simulink model "ExtraCredit"  (R2016a)
settings: Solver=VariableStepAuto  StartTime=0.0  StopTime=10.0  RelTol=1e-3
libraries: hdlsllib x17
(part 1 of 2)
settings Model: Creator=duyvu  LastModifiedBy=duyvu

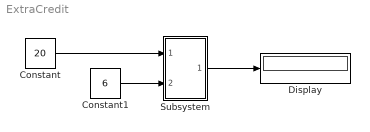
== system ExtraCredit ==
  Constant : Constant  Value=20  OutDataTypeStr=int8
  Constant1 : Constant  Value=6  OutDataTypeStr=int8
  Display : Display
  Subsystem : Subsystem
  wires:
  Subsystem/1(Result) -> Display/1
  Constant/1 -> Subsystem/1(Number1)
  Constant1/1 -> Subsystem/2(Number2)

== system ExtraCredit/Subsystem ==
  Number1 : Inport  OutDataTypeStr=int8
  Number2 : Inport  Port=2  OutDataTypeStr=int8
  Subsystem : Subsystem
  Result : Outport  OutDataTypeStr=int16
  wires:
  Number1/1 -> Subsystem/1(Number1)
  Number2/1 -> Subsystem/2(Number2)
  Subsystem/1(Result) -> Result/1

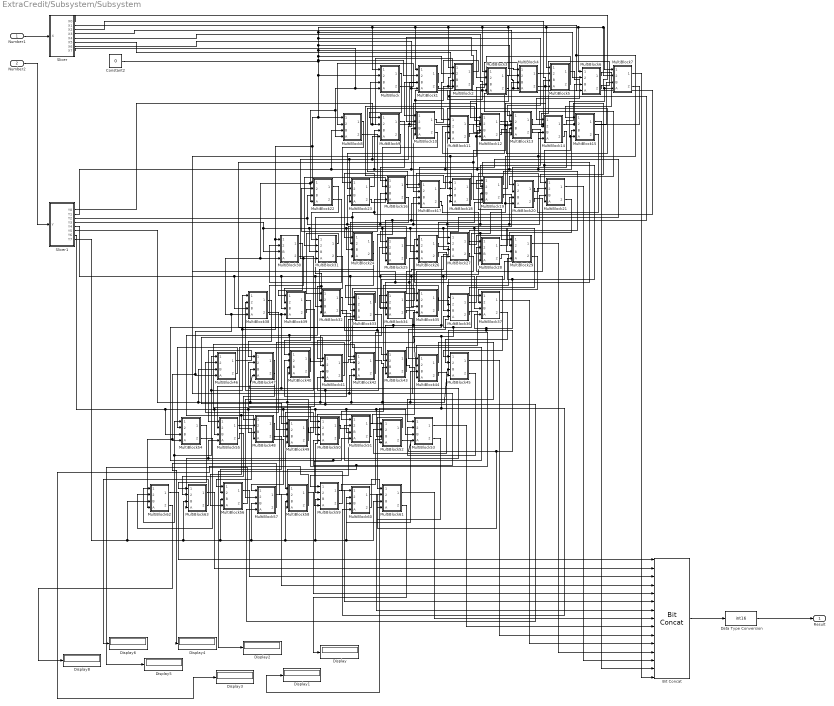
== system ExtraCredit/Subsystem/Subsystem ==
  Number1 : Inport  OutDataTypeStr=int8
  Number2 : Inport  Port=2  OutDataTypeStr=int8
  Bit Concat : hdlsllib/HDL Operations/Bit Concat  numInputs=15
  Constant2 : Constant  Value=0  OutDataTypeStr=boolean
  Data Type Conversion : DataTypeConversion  OutDataTypeStr=int16  ConvertRealWorld=Stored Integer (SI)
  Display{,1..6,8} (8 alike) : Display
      Display settings: Format=binary (Stored Integer)
      Display1 settings: Format=binary (Stored Integer)
  MultiBlock : Subsystem
  MultiBlock1 : Subsystem
  MultiBlock10 : Subsystem
  MultiBlock11 : Subsystem
  MultiBlock12 : Subsystem
  MultiBlock13 : Subsystem
  MultiBlock14 : Subsystem
  MultiBlock15 : Subsystem
  MultiBlock16 : Subsystem
  MultiBlock17 : Subsystem
  MultiBlock18 : Subsystem
  MultiBlock19 : Subsystem
  MultiBlock2 : Subsystem
  MultiBlock20 : Subsystem
  MultiBlock21 : Subsystem
  MultiBlock22 : Subsystem
  MultiBlock23 : Subsystem
  MultiBlock24 : Subsystem
  MultiBlock25 : Subsystem
  MultiBlock26 : Subsystem
  MultiBlock27 : Subsystem
  MultiBlock28 : Subsystem
  MultiBlock29 : Subsystem
  MultiBlock3 : Subsystem
  MultiBlock30 : Subsystem
  MultiBlock31 : Subsystem
  MultiBlock32 : Subsystem
  MultiBlock33 : Subsystem
  MultiBlock34 : Subsystem
  MultiBlock35 : Subsystem
  MultiBlock36 : Subsystem
  MultiBlock37 : Subsystem
  MultiBlock38 : Subsystem
  MultiBlock39 : Subsystem
  MultiBlock4 : Subsystem
  MultiBlock40 : Subsystem
  MultiBlock41 : Subsystem
  MultiBlock42 : Subsystem
  MultiBlock43 : Subsystem
  MultiBlock44 : Subsystem
  MultiBlock45 : Subsystem
  MultiBlock46 : Subsystem
  MultiBlock47 : Subsystem
  MultiBlock48 : Subsystem
  MultiBlock49 : Subsystem
  MultiBlock5 : Subsystem
  MultiBlock50 : Subsystem
  MultiBlock51 : Subsystem
  MultiBlock52 : Subsystem
  MultiBlock53 : Subsystem
  MultiBlock54 : Subsystem
  MultiBlock55 : Subsystem
  MultiBlock56 : Subsystem
  MultiBlock57 : Subsystem
  MultiBlock58 : Subsystem
  MultiBlock59 : Subsystem
  MultiBlock6 : Subsystem
  MultiBlock60 : Subsystem
  MultiBlock61 : Subsystem
  MultiBlock62 : Subsystem
  MultiBlock63 : Subsystem
  MultiBlock7 : Subsystem
  MultiBlock8 : Subsystem
  MultiBlock9 : Subsystem
  Slicer : Subsystem
  Slicer1 : Subsystem
  Result : Outport  OutDataTypeStr=int16
  wires:
  MultiBlock15/2(Carry) -> MultiBlock21/2(Cin)
  MultiBlock3/1(Sum) -> MultiBlock12/1(SumIn)
  Slicer1/1(Y0) -> MultiBlock/3(B), MultiBlock1/3(B), MultiBlock2/3(B), MultiBlock3/3(B), MultiBlock4/3(B), MultiBlock5/3(B), MultiBlock6/3(B), MultiBlock7/3(B)
  MultiBlock6/1(Sum) -> MultiBlock15/1(SumIn)
  MultiBlock12/1(Sum) -> MultiBlock19/1(SumIn)
  MultiBlock5/1(Sum) -> MultiBlock14/1(SumIn)
  MultiBlock/1(Sum) -> MultiBlock9/1(SumIn)
  MultiBlock4/1(Sum) -> MultiBlock13/1(SumIn)
  MultiBlock2/2(Carry) -> MultiBlock10/2(Cin)
  MultiBlock10/2(Carry) -> MultiBlock16/2(Cin)
  MultiBlock2/1(Sum) -> MultiBlock11/1(SumIn)
  MultiBlock1/1(Sum) -> MultiBlock10/1(SumIn)
  MultiBlock12/2(Carry) -> MultiBlock18/2(Cin)
  MultiBlock62/1(Sum) -> Bit Concat/1
  MultiBlock60/1(Sum) -> Bit Concat/7
  MultiBlock13/2(Carry) -> MultiBlock19/2(Cin)
  MultiBlock14/2(Carry) -> MultiBlock20/2(Cin)
  MultiBlock63/1(Sum) -> Bit Concat/2
  MultiBlock6/2(Carry) -> MultiBlock14/2(Cin)
  MultiBlock58/1(Sum) -> Bit Concat/5
  MultiBlock56/1(Sum) -> Bit Concat/3
  MultiBlock5/2(Carry) -> MultiBlock13/2(Cin)
  MultiBlock15/1(Sum) -> Bit Concat/14
  Slicer1/7(Y6) -> MultiBlock54/3(B), MultiBlock55/3(B), MultiBlock48/3(B), MultiBlock49/3(B), MultiBlock50/3(B), MultiBlock51/3(B), MultiBlock52/3(B), MultiBlock53/3(B)
  MultiBlock4/2(Carry) -> MultiBlock12/2(Cin)
  MultiBlock7/2(Carry) -> MultiBlock15/2(Cin)
  MultiBlock52/2(Carry) -> MultiBlock60/2(Cin)
  MultiBlock21/2(Carry) -> MultiBlock29/2(Cin)
  MultiBlock49/2(Carry) -> MultiBlock57/2(Cin)
  MultiBlock34/2(Carry) -> MultiBlock42/2(Cin)
  MultiBlock42/2(Carry) -> MultiBlock50/2(Cin)
  MultiBlock33/2(Carry) -> MultiBlock41/2(Cin)
  MultiBlock22/1(Sum) -> MultiBlock31/1(SumIn)
  MultiBlock16/1(Sum) -> MultiBlock25/1(SumIn)
  MultiBlock32/2(Carry) -> MultiBlock40/2(Cin)
  MultiBlock41/2(Carry) -> MultiBlock49/2(Cin)
  MultiBlock39/2(Carry) -> MultiBlock47/2(Cin)
  MultiBlock57/2(Carry) -> Display4/1
  MultiBlock30/1(Sum) -> MultiBlock39/1(SumIn)
  MultiBlock31/1(Sum) -> MultiBlock32/1(SumIn)
  MultiBlock55/2(Carry) -> MultiBlock63/2(Cin)
  MultiBlock24/2(Carry) -> MultiBlock32/2(Cin)
  MultiBlock59/2(Carry) -> Display2/1
  MultiBlock20/2(Carry) -> MultiBlock28/2(Cin)
  MultiBlock31/2(Carry) -> MultiBlock39/2(Cin)
  MultiBlock28/1(Sum) -> MultiBlock37/1(SumIn)
  MultiBlock36/1(Sum) -> MultiBlock45/1(SumIn)
  MultiBlock25/2(Carry) -> MultiBlock33/2(Cin)
  MultiBlock34/1(Sum) -> MultiBlock43/1(SumIn)
  MultiBlock45/2(Carry) -> MultiBlock53/2(Cin)
  MultiBlock10/1(Sum) -> MultiBlock17/1(SumIn)
  MultiBlock61/2(Carry) -> Display/1
  MultiBlock38/2(Carry) -> MultiBlock46/2(Cin)
  MultiBlock17/2(Carry) -> MultiBlock25/2(Cin)
  MultiBlock19/2(Carry) -> MultiBlock27/2(Cin)
  MultiBlock43/1(Sum) -> MultiBlock52/1(SumIn)
  MultiBlock44/1(Sum) -> MultiBlock53/1(SumIn)
  MultiBlock52/1(Sum) -> MultiBlock61/1(SumIn)
  MultiBlock46/2(Carry) -> MultiBlock54/2(Cin)
  MultiBlock47/2(Carry) -> MultiBlock55/2(Cin)
  MultiBlock9/1(Sum) -> MultiBlock16/1(SumIn)
  MultiBlock18/2(Carry) -> MultiBlock26/2(Cin)
  MultiBlock56/2(Carry) -> Display5/1
  MultiBlock8/1(Sum) -> MultiBlock23/1(SumIn)
  MultiBlock32/1(Sum) -> MultiBlock41/1(SumIn)
  MultiBlock58/2(Carry) -> Display3/1
  MultiBlock35/1(Sum) -> MultiBlock44/1(SumIn)
  MultiBlock51/2(Carry) -> MultiBlock59/2(Cin)
  MultiBlock16/2(Carry) -> MultiBlock24/2(Cin)
  MultiBlock30/2(Carry) -> MultiBlock38/2(Cin)
  MultiBlock22/2(Carry) -> MultiBlock30/2(Cin)
  MultiBlock47/1(Sum) -> MultiBlock48/1(SumIn)
  MultiBlock44/2(Carry) -> MultiBlock52/2(Cin)
  MultiBlock50/2(Carry) -> MultiBlock58/2(Cin)
  MultiBlock39/1(Sum) -> MultiBlock40/1(SumIn)
  MultiBlock41/1(Sum) -> MultiBlock50/1(SumIn)
  MultiBlock42/1(Sum) -> MultiBlock51/1(SumIn)
  MultiBlock37/2(Carry) -> MultiBlock45/2(Cin)
  MultiBlock50/1(Sum) -> MultiBlock59/1(SumIn)
  MultiBlock23/2(Carry) -> MultiBlock31/2(Cin)
  MultiBlock25/1(Sum) -> MultiBlock34/1(SumIn)
  MultiBlock27/1(Sum) -> MultiBlock36/1(SumIn)
  MultiBlock38/1(Sum) -> MultiBlock47/1(SumIn)
  MultiBlock20/1(Sum) -> MultiBlock29/1(SumIn)
  MultiBlock18/1(Sum) -> MultiBlock27/1(SumIn)
  MultiBlock19/1(Sum) -> MultiBlock28/1(SumIn)
  MultiBlock17/1(Sum) -> MultiBlock26/1(SumIn)
  MultiBlock24/1(Sum) -> MultiBlock33/1(SumIn)
  MultiBlock35/2(Carry) -> MultiBlock43/2(Cin)
  MultiBlock43/2(Carry) -> MultiBlock51/2(Cin)
  MultiBlock54/1(Sum) -> MultiBlock63/1(SumIn)
  MultiBlock40/1(Sum) -> MultiBlock49/1(SumIn)
  MultiBlock54/2(Carry) -> MultiBlock62/2(Cin)
  MultiBlock40/2(Carry) -> MultiBlock48/2(Cin)
  MultiBlock55/1(Sum) -> MultiBlock56/1(SumIn)
  MultiBlock48/2(Carry) -> MultiBlock56/2(Cin)
  MultiBlock51/1(Sum) -> MultiBlock60/1(SumIn)
  MultiBlock26/1(Sum) -> MultiBlock35/1(SumIn)
  MultiBlock53/2(Carry) -> MultiBlock61/2(Cin)
  MultiBlock33/1(Sum) -> MultiBlock42/1(SumIn)
  Slicer/8(X7) -> MultiBlock30/4(A), MultiBlock62/4(A), MultiBlock54/4(A), MultiBlock46/4(A), MultiBlock38/4(A), MultiBlock22/4(A), MultiBlock8/4(A), MultiBlock/4(A)
  Slicer/4(X3) -> MultiBlock26/4(A), MultiBlock58/4(A), MultiBlock50/4(A), MultiBlock42/4(A), MultiBlock34/4(A), MultiBlock18/4(A), MultiBlock12/4(A), MultiBlock4/4(A)
  Slicer/5(X4) -> MultiBlock33/4(A), MultiBlock49/4(A), MultiBlock57/4(A), MultiBlock41/4(A), MultiBlock25/4(A), MultiBlock17/4(A), MultiBlock11/4(A), MultiBlock3/4(A)
  MultiBlock36/2(Carry) -> MultiBlock44/2(Cin)
  MultiBlock46/1(Sum) -> MultiBlock55/1(SumIn)
  Slicer1/4(Y3) -> MultiBlock30/3(B), MultiBlock31/3(B), MultiBlock24/3(B), MultiBlock25/3(B), MultiBlock26/3(B), MultiBlock27/3(B), MultiBlock28/3(B), MultiBlock29/3(B)
  Slicer/3(X2) -> MultiBlock5/4(A), MultiBlock19/4(A), MultiBlock27/4(A), MultiBlock59/4(A), MultiBlock51/4(A), MultiBlock43/4(A), MultiBlock35/4(A), MultiBlock13/4(A)
  Slicer/6(X5) -> MultiBlock56/4(A), MultiBlock48/4(A), MultiBlock40/4(A), MultiBlock32/4(A), MultiBlock24/4(A), MultiBlock16/4(A), MultiBlock10/4(A), MultiBlock2/4(A)
  Slicer/1(X0) -> MultiBlock45/4(A), MultiBlock61/4(A), MultiBlock53/4(A), MultiBlock37/4(A), MultiBlock29/4(A), MultiBlock21/4(A), MultiBlock15/4(A), MultiBlock7/4(A)
  Slicer/7(X6) -> MultiBlock47/4(A), MultiBlock63/4(A), MultiBlock55/4(A), MultiBlock39/4(A), MultiBlock31/4(A), MultiBlock23/4(A), MultiBlock9/4(A), MultiBlock1/4(A)
  Slicer/2(X1) -> MultiBlock6/4(A), MultiBlock44/4(A), MultiBlock52/4(A), MultiBlock60/4(A), MultiBlock36/4(A), MultiBlock28/4(A), MultiBlock20/4(A), MultiBlock14/4(A)
  MultiBlock26/2(Carry) -> MultiBlock34/2(Cin)
  Slicer1/6(Y5) -> MultiBlock46/3(B), MultiBlock47/3(B), MultiBlock40/3(B), MultiBlock41/3(B), MultiBlock42/3(B), MultiBlock43/3(B), MultiBlock44/3(B), MultiBlock45/3(B)
  MultiBlock13/1(Sum) -> MultiBlock20/1(SumIn)
  MultiBlock8/2(Carry) -> MultiBlock22/2(Cin)
  Slicer1/3(Y2) -> MultiBlock23/3(B), MultiBlock18/3(B), MultiBlock19/3(B), MultiBlock20/3(B), MultiBlock21/3(B), MultiBlock17/3(B), MultiBlock16/3(B), MultiBlock22/3(B)
  Number1/1 -> Slicer/1(X)
  Number2/1 -> Slicer1/1(Y)
  Slicer1/2(Y1) -> MultiBlock9/3(B), MultiBlock10/3(B), MultiBlock11/3(B), MultiBlock12/3(B), MultiBlock13/3(B), MultiBlock14/3(B), MultiBlock15/3(B), MultiBlock8/3(B)
  MultiBlock29/1(Sum) -> Bit Concat/12
  MultiBlock61/1(Sum) -> Bit Concat/8
  MultiBlock21/1(Sum) -> Bit Concat/13
  MultiBlock28/2(Carry) -> MultiBlock36/2(Cin)
  MultiBlock27/2(Carry) -> MultiBlock35/2(Cin)
  MultiBlock29/2(Carry) -> MultiBlock37/2(Cin)
  MultiBlock37/1(Sum) -> Bit Concat/11
  Constant2/1 -> MultiBlock/1(SumIn), MultiBlock1/1(SumIn), MultiBlock6/1(SumIn), MultiBlock7/1(SumIn), MultiBlock7/2(Cin), MultiBlock5/1(SumIn), MultiBlock4/1(SumIn), MultiBlock3/1(SumIn), MultiBlock2/1(SumIn), MultiBlock6/2(Cin), MultiBlock5/2(Cin), MultiBlock4/2(Cin), MultiBlock3/2(Cin), MultiBlock2/2(Cin), MultiBlock1/2(Cin), MultiBlock38/1(SumIn), MultiBlock46/1(SumIn), MultiBlock54/1(SumIn), MultiBlock62/1(SumIn), MultiBlock30/1(SumIn), MultiBlock22/1(SumIn), MultiBlock8/1(SumIn), MultiBlock/2(Cin)
  MultiBlock53/1(Sum) -> Bit Concat/9
  MultiBlock45/1(Sum) -> Bit Concat/10
  MultiBlock23/1(Sum) -> MultiBlock24/1(SumIn)
  MultiBlock59/1(Sum) -> Bit Concat/6
  Slicer1/8(Y7) -> MultiBlock62/3(B), MultiBlock63/3(B), MultiBlock56/3(B), MultiBlock57/3(B), MultiBlock58/3(B), MultiBlock59/3(B), MultiBlock61/3(B), MultiBlock60/3(B)
  MultiBlock48/1(Sum) -> MultiBlock57/1(SumIn)
  MultiBlock57/1(Sum) -> Bit Concat/4
  MultiBlock62/2(Carry) -> Display8/1
  Bit Concat/1 -> Data Type Conversion/1
  MultiBlock/2(Carry) -> MultiBlock8/2(Cin)
  Data Type Conversion/1 -> Result/1
  MultiBlock49/1(Sum) -> MultiBlock58/1(SumIn)
  MultiBlock63/2(Carry) -> Display6/1
  MultiBlock3/2(Carry) -> MultiBlock11/2(Cin)
  MultiBlock1/2(Carry) -> MultiBlock9/2(Cin)
  Slicer1/5(Y4) -> MultiBlock38/3(B), MultiBlock39/3(B), MultiBlock32/3(B), MultiBlock33/3(B), MultiBlock34/3(B), MultiBlock35/3(B), MultiBlock36/3(B), MultiBlock37/3(B)
  MultiBlock60/2(Carry) -> Display1/1
  MultiBlock7/1(Sum) -> Bit Concat/15
  MultiBlock11/2(Carry) -> MultiBlock17/2(Cin)
  MultiBlock9/2(Carry) -> MultiBlock23/2(Cin)
  MultiBlock11/1(Sum) -> MultiBlock18/1(SumIn)
  MultiBlock14/1(Sum) -> MultiBlock21/1(SumIn)

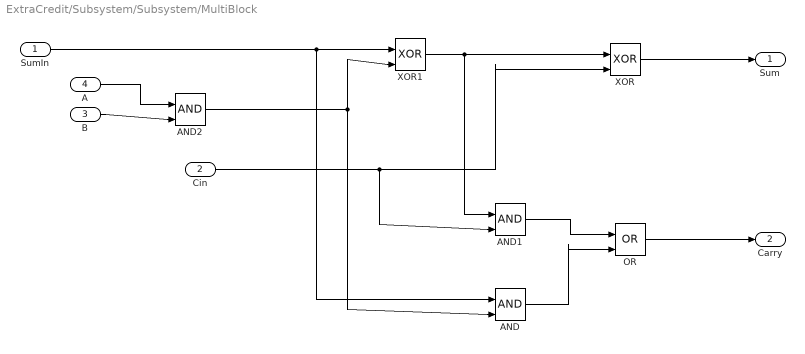
== system ExtraCredit/Subsystem/Subsystem/MultiBlock ==
  SumIn : Inport
  Cin : Inport  Port=2
  B : Inport  Port=3
  A : Inport  Port=4
  AND : Logic  IconShape=distinctive  AllPortsSameDT=off  OutDataTypeStr=boolean
  AND1 : Logic  IconShape=distinctive  AllPortsSameDT=off  OutDataTypeStr=boolean
  AND2 : Logic  IconShape=distinctive  AllPortsSameDT=off  OutDataTypeStr=boolean
  "OR " : Logic  Operator=OR  IconShape=distinctive  AllPortsSameDT=off  OutDataTypeStr=boolean
  XOR : Logic  Operator=XOR  IconShape=distinctive  AllPortsSameDT=off  OutDataTypeStr=boolean
  XOR1 : Logic  Operator=XOR  IconShape=distinctive  AllPortsSameDT=off  OutDataTypeStr=boolean
  Sum : Outport
  Carry : Outport  Port=2
  wires:
  SumIn/1 -> XOR1/1, AND/1
  XOR1/1 -> AND1/1, XOR/1
  Cin/1 -> XOR/2, AND1/2
  XOR/1 -> Sum/1
  AND2/1 -> AND/2, XOR1/2
  "OR "/1 -> Carry/1
  AND1/1 -> "OR "/1
  AND/1 -> "OR "/2
  B/1 -> AND2/2
  A/1 -> AND2/1

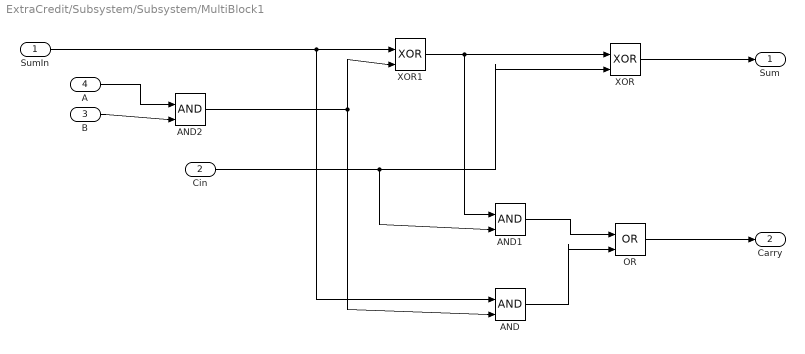
== system ExtraCredit/Subsystem/Subsystem/MultiBlock1 ==
  SumIn : Inport
  Cin : Inport  Port=2
  B : Inport  Port=3
  A : Inport  Port=4
  AND : Logic  IconShape=distinctive  AllPortsSameDT=off  OutDataTypeStr=boolean
  AND1 : Logic  IconShape=distinctive  AllPortsSameDT=off  OutDataTypeStr=boolean
  AND2 : Logic  IconShape=distinctive  AllPortsSameDT=off  OutDataTypeStr=boolean
  "OR " : Logic  Operator=OR  IconShape=distinctive  AllPortsSameDT=off  OutDataTypeStr=boolean
  XOR : Logic  Operator=XOR  IconShape=distinctive  AllPortsSameDT=off  OutDataTypeStr=boolean
  XOR1 : Logic  Operator=XOR  IconShape=distinctive  AllPortsSameDT=off  OutDataTypeStr=boolean
  Sum : Outport
  Carry : Outport  Port=2
  wires:
  SumIn/1 -> XOR1/1, AND/1
  XOR1/1 -> AND1/1, XOR/1
  Cin/1 -> XOR/2, AND1/2
  XOR/1 -> Sum/1
  AND2/1 -> AND/2, XOR1/2
  "OR "/1 -> Carry/1
  AND1/1 -> "OR "/1
  AND/1 -> "OR "/2
  B/1 -> AND2/2
  A/1 -> AND2/1

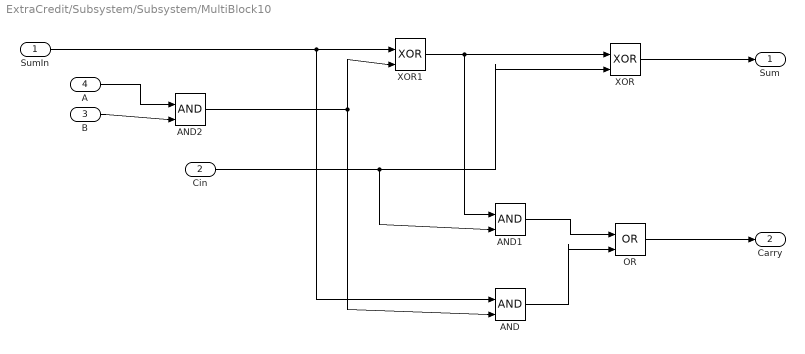
== system ExtraCredit/Subsystem/Subsystem/MultiBlock10 ==
  SumIn : Inport
  Cin : Inport  Port=2
  B : Inport  Port=3
  A : Inport  Port=4
  AND : Logic  IconShape=distinctive  AllPortsSameDT=off  OutDataTypeStr=boolean
  AND1 : Logic  IconShape=distinctive  AllPortsSameDT=off  OutDataTypeStr=boolean
  AND2 : Logic  IconShape=distinctive  AllPortsSameDT=off  OutDataTypeStr=boolean
  "OR " : Logic  Operator=OR  IconShape=distinctive  AllPortsSameDT=off  OutDataTypeStr=boolean
  XOR : Logic  Operator=XOR  IconShape=distinctive  AllPortsSameDT=off  OutDataTypeStr=boolean
  XOR1 : Logic  Operator=XOR  IconShape=distinctive  AllPortsSameDT=off  OutDataTypeStr=boolean
  Sum : Outport
  Carry : Outport  Port=2
  wires:
  SumIn/1 -> XOR1/1, AND/1
  XOR1/1 -> AND1/1, XOR/1
  Cin/1 -> XOR/2, AND1/2
  XOR/1 -> Sum/1
  AND2/1 -> AND/2, XOR1/2
  "OR "/1 -> Carry/1
  AND1/1 -> "OR "/1
  AND/1 -> "OR "/2
  B/1 -> AND2/2
  A/1 -> AND2/1

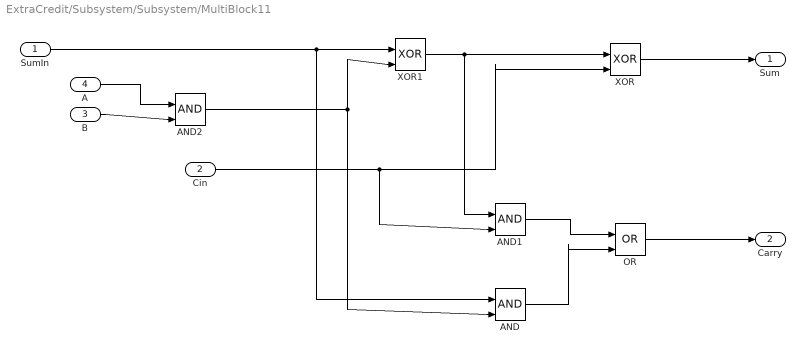
== system ExtraCredit/Subsystem/Subsystem/MultiBlock11 ==
  SumIn : Inport
  Cin : Inport  Port=2
  B : Inport  Port=3
  A : Inport  Port=4
  AND : Logic  IconShape=distinctive  AllPortsSameDT=off  OutDataTypeStr=boolean
  AND1 : Logic  IconShape=distinctive  AllPortsSameDT=off  OutDataTypeStr=boolean
  AND2 : Logic  IconShape=distinctive  AllPortsSameDT=off  OutDataTypeStr=boolean
  "OR " : Logic  Operator=OR  IconShape=distinctive  AllPortsSameDT=off  OutDataTypeStr=boolean
  XOR : Logic  Operator=XOR  IconShape=distinctive  AllPortsSameDT=off  OutDataTypeStr=boolean
  XOR1 : Logic  Operator=XOR  IconShape=distinctive  AllPortsSameDT=off  OutDataTypeStr=boolean
  Sum : Outport
  Carry : Outport  Port=2
  wires:
  SumIn/1 -> XOR1/1, AND/1
  XOR1/1 -> AND1/1, XOR/1
  Cin/1 -> XOR/2, AND1/2
  XOR/1 -> Sum/1
  AND2/1 -> AND/2, XOR1/2
  "OR "/1 -> Carry/1
  AND1/1 -> "OR "/1
  AND/1 -> "OR "/2
  B/1 -> AND2/2
  A/1 -> AND2/1

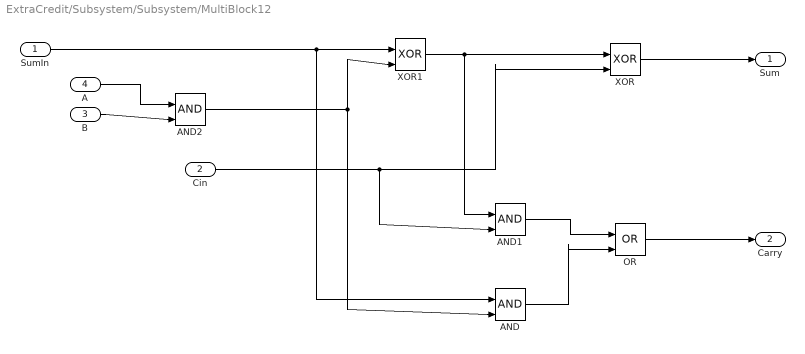
== system ExtraCredit/Subsystem/Subsystem/MultiBlock12 ==
  SumIn : Inport
  Cin : Inport  Port=2
  B : Inport  Port=3
  A : Inport  Port=4
  AND : Logic  IconShape=distinctive  AllPortsSameDT=off  OutDataTypeStr=boolean
  AND1 : Logic  IconShape=distinctive  AllPortsSameDT=off  OutDataTypeStr=boolean
  AND2 : Logic  IconShape=distinctive  AllPortsSameDT=off  OutDataTypeStr=boolean
  "OR " : Logic  Operator=OR  IconShape=distinctive  AllPortsSameDT=off  OutDataTypeStr=boolean
  XOR : Logic  Operator=XOR  IconShape=distinctive  AllPortsSameDT=off  OutDataTypeStr=boolean
  XOR1 : Logic  Operator=XOR  IconShape=distinctive  AllPortsSameDT=off  OutDataTypeStr=boolean
  Sum : Outport
  Carry : Outport  Port=2
  wires:
  SumIn/1 -> XOR1/1, AND/1
  XOR1/1 -> AND1/1, XOR/1
  Cin/1 -> XOR/2, AND1/2
  XOR/1 -> Sum/1
  AND2/1 -> AND/2, XOR1/2
  "OR "/1 -> Carry/1
  AND1/1 -> "OR "/1
  AND/1 -> "OR "/2
  B/1 -> AND2/2
  A/1 -> AND2/1

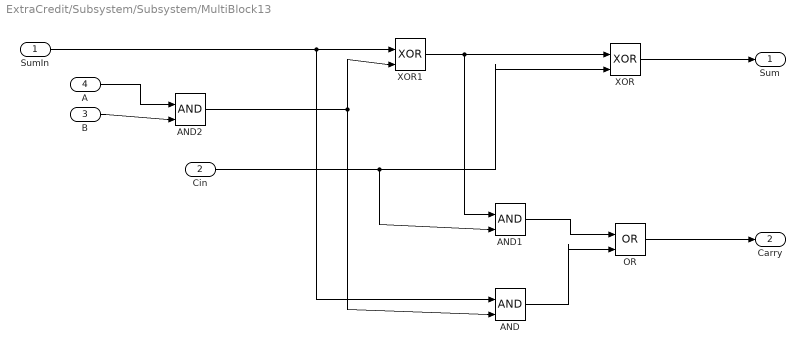
== system ExtraCredit/Subsystem/Subsystem/MultiBlock13 ==
  SumIn : Inport
  Cin : Inport  Port=2
  B : Inport  Port=3
  A : Inport  Port=4
  AND : Logic  IconShape=distinctive  AllPortsSameDT=off  OutDataTypeStr=boolean
  AND1 : Logic  IconShape=distinctive  AllPortsSameDT=off  OutDataTypeStr=boolean
  AND2 : Logic  IconShape=distinctive  AllPortsSameDT=off  OutDataTypeStr=boolean
  "OR " : Logic  Operator=OR  IconShape=distinctive  AllPortsSameDT=off  OutDataTypeStr=boolean
  XOR : Logic  Operator=XOR  IconShape=distinctive  AllPortsSameDT=off  OutDataTypeStr=boolean
  XOR1 : Logic  Operator=XOR  IconShape=distinctive  AllPortsSameDT=off  OutDataTypeStr=boolean
  Sum : Outport
  Carry : Outport  Port=2
  wires:
  SumIn/1 -> XOR1/1, AND/1
  XOR1/1 -> AND1/1, XOR/1
  Cin/1 -> XOR/2, AND1/2
  XOR/1 -> Sum/1
  AND2/1 -> AND/2, XOR1/2
  "OR "/1 -> Carry/1
  AND1/1 -> "OR "/1
  AND/1 -> "OR "/2
  B/1 -> AND2/2
  A/1 -> AND2/1

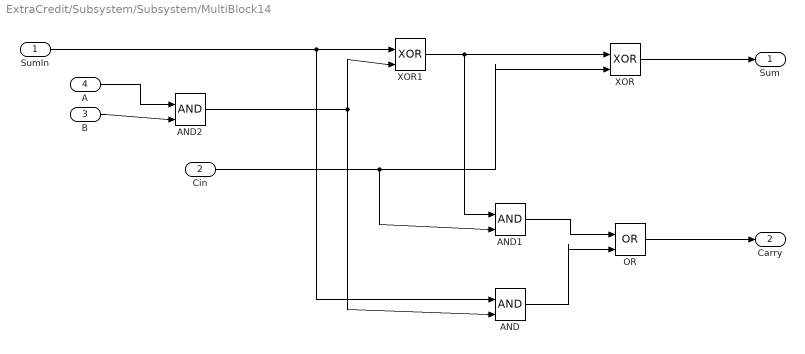
== system ExtraCredit/Subsystem/Subsystem/MultiBlock14 ==
  SumIn : Inport
  Cin : Inport  Port=2
  B : Inport  Port=3
  A : Inport  Port=4
  AND : Logic  IconShape=distinctive  AllPortsSameDT=off  OutDataTypeStr=boolean
  AND1 : Logic  IconShape=distinctive  AllPortsSameDT=off  OutDataTypeStr=boolean
  AND2 : Logic  IconShape=distinctive  AllPortsSameDT=off  OutDataTypeStr=boolean
  "OR " : Logic  Operator=OR  IconShape=distinctive  AllPortsSameDT=off  OutDataTypeStr=boolean
  XOR : Logic  Operator=XOR  IconShape=distinctive  AllPortsSameDT=off  OutDataTypeStr=boolean
  XOR1 : Logic  Operator=XOR  IconShape=distinctive  AllPortsSameDT=off  OutDataTypeStr=boolean
  Sum : Outport
  Carry : Outport  Port=2
  wires:
  SumIn/1 -> XOR1/1, AND/1
  XOR1/1 -> AND1/1, XOR/1
  Cin/1 -> XOR/2, AND1/2
  XOR/1 -> Sum/1
  AND2/1 -> AND/2, XOR1/2
  "OR "/1 -> Carry/1
  AND1/1 -> "OR "/1
  AND/1 -> "OR "/2
  B/1 -> AND2/2
  A/1 -> AND2/1

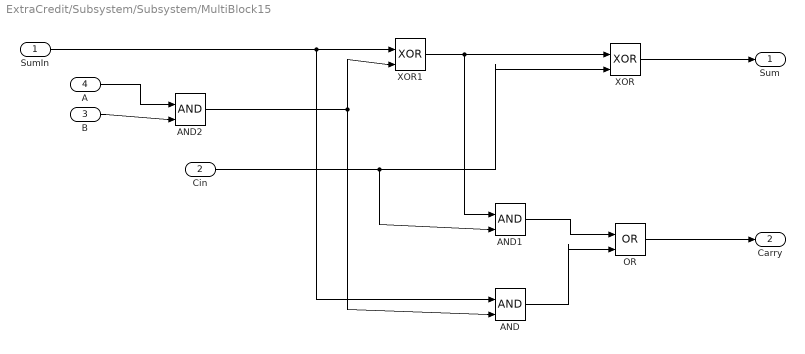
== system ExtraCredit/Subsystem/Subsystem/MultiBlock15 ==
  SumIn : Inport
  Cin : Inport  Port=2
  B : Inport  Port=3
  A : Inport  Port=4
  AND : Logic  IconShape=distinctive  AllPortsSameDT=off  OutDataTypeStr=boolean
  AND1 : Logic  IconShape=distinctive  AllPortsSameDT=off  OutDataTypeStr=boolean
  AND2 : Logic  IconShape=distinctive  AllPortsSameDT=off  OutDataTypeStr=boolean
  "OR " : Logic  Operator=OR  IconShape=distinctive  AllPortsSameDT=off  OutDataTypeStr=boolean
  XOR : Logic  Operator=XOR  IconShape=distinctive  AllPortsSameDT=off  OutDataTypeStr=boolean
  XOR1 : Logic  Operator=XOR  IconShape=distinctive  AllPortsSameDT=off  OutDataTypeStr=boolean
  Sum : Outport
  Carry : Outport  Port=2
  wires:
  SumIn/1 -> XOR1/1, AND/1
  XOR1/1 -> AND1/1, XOR/1
  Cin/1 -> XOR/2, AND1/2
  XOR/1 -> Sum/1
  AND2/1 -> AND/2, XOR1/2
  "OR "/1 -> Carry/1
  AND1/1 -> "OR "/1
  AND/1 -> "OR "/2
  B/1 -> AND2/2
  A/1 -> AND2/1

== system ExtraCredit/Subsystem/Subsystem/MultiBlock16 ==
  SumIn : Inport
  Cin : Inport  Port=2
  B : Inport  Port=3
  A : Inport  Port=4
  AND : Logic  IconShape=distinctive  AllPortsSameDT=off  OutDataTypeStr=boolean
  AND1 : Logic  IconShape=distinctive  AllPortsSameDT=off  OutDataTypeStr=boolean
  AND2 : Logic  IconShape=distinctive  AllPortsSameDT=off  OutDataTypeStr=boolean
  "OR " : Logic  Operator=OR  IconShape=distinctive  AllPortsSameDT=off  OutDataTypeStr=boolean
  XOR : Logic  Operator=XOR  IconShape=distinctive  AllPortsSameDT=off  OutDataTypeStr=boolean
  XOR1 : Logic  Operator=XOR  IconShape=distinctive  AllPortsSameDT=off  OutDataTypeStr=boolean
  Sum : Outport
  Carry : Outport  Port=2
  wires:
  SumIn/1 -> XOR1/1, AND/1
  XOR1/1 -> AND1/1, XOR/1
  Cin/1 -> XOR/2, AND1/2
  XOR/1 -> Sum/1
  AND2/1 -> AND/2, XOR1/2
  "OR "/1 -> Carry/1
  AND1/1 -> "OR "/1
  AND/1 -> "OR "/2
  B/1 -> AND2/2
  A/1 -> AND2/1

== system ExtraCredit/Subsystem/Subsystem/MultiBlock17 ==
  SumIn : Inport
  Cin : Inport  Port=2
  B : Inport  Port=3
  A : Inport  Port=4
  AND : Logic  IconShape=distinctive  AllPortsSameDT=off  OutDataTypeStr=boolean
  AND1 : Logic  IconShape=distinctive  AllPortsSameDT=off  OutDataTypeStr=boolean
  AND2 : Logic  IconShape=distinctive  AllPortsSameDT=off  OutDataTypeStr=boolean
  "OR " : Logic  Operator=OR  IconShape=distinctive  AllPortsSameDT=off  OutDataTypeStr=boolean
  XOR : Logic  Operator=XOR  IconShape=distinctive  AllPortsSameDT=off  OutDataTypeStr=boolean
  XOR1 : Logic  Operator=XOR  IconShape=distinctive  AllPortsSameDT=off  OutDataTypeStr=boolean
  Sum : Outport
  Carry : Outport  Port=2
  wires:
  SumIn/1 -> XOR1/1, AND/1
  XOR1/1 -> AND1/1, XOR/1
  Cin/1 -> XOR/2, AND1/2
  XOR/1 -> Sum/1
  AND2/1 -> AND/2, XOR1/2
  "OR "/1 -> Carry/1
  AND1/1 -> "OR "/1
  AND/1 -> "OR "/2
  B/1 -> AND2/2
  A/1 -> AND2/1

== system ExtraCredit/Subsystem/Subsystem/MultiBlock18 ==
  SumIn : Inport
  Cin : Inport  Port=2
  B : Inport  Port=3
  A : Inport  Port=4
  AND : Logic  IconShape=distinctive  AllPortsSameDT=off  OutDataTypeStr=boolean
  AND1 : Logic  IconShape=distinctive  AllPortsSameDT=off  OutDataTypeStr=boolean
  AND2 : Logic  IconShape=distinctive  AllPortsSameDT=off  OutDataTypeStr=boolean
  "OR " : Logic  Operator=OR  IconShape=distinctive  AllPortsSameDT=off  OutDataTypeStr=boolean
  XOR : Logic  Operator=XOR  IconShape=distinctive  AllPortsSameDT=off  OutDataTypeStr=boolean
  XOR1 : Logic  Operator=XOR  IconShape=distinctive  AllPortsSameDT=off  OutDataTypeStr=boolean
  Sum : Outport
  Carry : Outport  Port=2
  wires:
  SumIn/1 -> XOR1/1, AND/1
  XOR1/1 -> AND1/1, XOR/1
  Cin/1 -> XOR/2, AND1/2
  XOR/1 -> Sum/1
  AND2/1 -> AND/2, XOR1/2
  "OR "/1 -> Carry/1
  AND1/1 -> "OR "/1
  AND/1 -> "OR "/2
  B/1 -> AND2/2
  A/1 -> AND2/1

== system ExtraCredit/Subsystem/Subsystem/MultiBlock19 ==
  SumIn : Inport
  Cin : Inport  Port=2
  B : Inport  Port=3
  A : Inport  Port=4
  AND : Logic  IconShape=distinctive  AllPortsSameDT=off  OutDataTypeStr=boolean
  AND1 : Logic  IconShape=distinctive  AllPortsSameDT=off  OutDataTypeStr=boolean
  AND2 : Logic  IconShape=distinctive  AllPortsSameDT=off  OutDataTypeStr=boolean
  "OR " : Logic  Operator=OR  IconShape=distinctive  AllPortsSameDT=off  OutDataTypeStr=boolean
  XOR : Logic  Operator=XOR  IconShape=distinctive  AllPortsSameDT=off  OutDataTypeStr=boolean
  XOR1 : Logic  Operator=XOR  IconShape=distinctive  AllPortsSameDT=off  OutDataTypeStr=boolean
  Sum : Outport
  Carry : Outport  Port=2
  wires:
  SumIn/1 -> XOR1/1, AND/1
  XOR1/1 -> AND1/1, XOR/1
  Cin/1 -> XOR/2, AND1/2
  XOR/1 -> Sum/1
  AND2/1 -> AND/2, XOR1/2
  "OR "/1 -> Carry/1
  AND1/1 -> "OR "/1
  AND/1 -> "OR "/2
  B/1 -> AND2/2
  A/1 -> AND2/1

== system ExtraCredit/Subsystem/Subsystem/MultiBlock2 ==
  SumIn : Inport
  Cin : Inport  Port=2
  B : Inport  Port=3
  A : Inport  Port=4
  AND : Logic  IconShape=distinctive  AllPortsSameDT=off  OutDataTypeStr=boolean
  AND1 : Logic  IconShape=distinctive  AllPortsSameDT=off  OutDataTypeStr=boolean
  AND2 : Logic  IconShape=distinctive  AllPortsSameDT=off  OutDataTypeStr=boolean
  "OR " : Logic  Operator=OR  IconShape=distinctive  AllPortsSameDT=off  OutDataTypeStr=boolean
  XOR : Logic  Operator=XOR  IconShape=distinctive  AllPortsSameDT=off  OutDataTypeStr=boolean
  XOR1 : Logic  Operator=XOR  IconShape=distinctive  AllPortsSameDT=off  OutDataTypeStr=boolean
  Sum : Outport
  Carry : Outport  Port=2
  wires:
  SumIn/1 -> XOR1/1, AND/1
  XOR1/1 -> AND1/1, XOR/1
  Cin/1 -> XOR/2, AND1/2
  XOR/1 -> Sum/1
  AND2/1 -> AND/2, XOR1/2
  "OR "/1 -> Carry/1
  AND1/1 -> "OR "/1
  AND/1 -> "OR "/2
  B/1 -> AND2/2
  A/1 -> AND2/1

== system ExtraCredit/Subsystem/Subsystem/MultiBlock20 ==
  SumIn : Inport
  Cin : Inport  Port=2
  B : Inport  Port=3
  A : Inport  Port=4
  AND : Logic  IconShape=distinctive  AllPortsSameDT=off  OutDataTypeStr=boolean
  AND1 : Logic  IconShape=distinctive  AllPortsSameDT=off  OutDataTypeStr=boolean
  AND2 : Logic  IconShape=distinctive  AllPortsSameDT=off  OutDataTypeStr=boolean
  "OR " : Logic  Operator=OR  IconShape=distinctive  AllPortsSameDT=off  OutDataTypeStr=boolean
  XOR : Logic  Operator=XOR  IconShape=distinctive  AllPortsSameDT=off  OutDataTypeStr=boolean
  XOR1 : Logic  Operator=XOR  IconShape=distinctive  AllPortsSameDT=off  OutDataTypeStr=boolean
  Sum : Outport
  Carry : Outport  Port=2
  wires:
  SumIn/1 -> XOR1/1, AND/1
  XOR1/1 -> AND1/1, XOR/1
  Cin/1 -> XOR/2, AND1/2
  XOR/1 -> Sum/1
  AND2/1 -> AND/2, XOR1/2
  "OR "/1 -> Carry/1
  AND1/1 -> "OR "/1
  AND/1 -> "OR "/2
  B/1 -> AND2/2
  A/1 -> AND2/1

== system ExtraCredit/Subsystem/Subsystem/MultiBlock21 ==
  SumIn : Inport
  Cin : Inport  Port=2
  B : Inport  Port=3
  A : Inport  Port=4
  AND : Logic  IconShape=distinctive  AllPortsSameDT=off  OutDataTypeStr=boolean
  AND1 : Logic  IconShape=distinctive  AllPortsSameDT=off  OutDataTypeStr=boolean
  AND2 : Logic  IconShape=distinctive  AllPortsSameDT=off  OutDataTypeStr=boolean
  "OR " : Logic  Operator=OR  IconShape=distinctive  AllPortsSameDT=off  OutDataTypeStr=boolean
  XOR : Logic  Operator=XOR  IconShape=distinctive  AllPortsSameDT=off  OutDataTypeStr=boolean
  XOR1 : Logic  Operator=XOR  IconShape=distinctive  AllPortsSameDT=off  OutDataTypeStr=boolean
  Sum : Outport
  Carry : Outport  Port=2
  wires:
  SumIn/1 -> XOR1/1, AND/1
  XOR1/1 -> AND1/1, XOR/1
  Cin/1 -> XOR/2, AND1/2
  XOR/1 -> Sum/1
  AND2/1 -> AND/2, XOR1/2
  "OR "/1 -> Carry/1
  AND1/1 -> "OR "/1
  AND/1 -> "OR "/2
  B/1 -> AND2/2
  A/1 -> AND2/1

== system ExtraCredit/Subsystem/Subsystem/MultiBlock22 ==
  SumIn : Inport
  Cin : Inport  Port=2
  B : Inport  Port=3
  A : Inport  Port=4
  AND : Logic  IconShape=distinctive  AllPortsSameDT=off  OutDataTypeStr=boolean
  AND1 : Logic  IconShape=distinctive  AllPortsSameDT=off  OutDataTypeStr=boolean
  AND2 : Logic  IconShape=distinctive  AllPortsSameDT=off  OutDataTypeStr=boolean
  "OR " : Logic  Operator=OR  IconShape=distinctive  AllPortsSameDT=off  OutDataTypeStr=boolean
  XOR : Logic  Operator=XOR  IconShape=distinctive  AllPortsSameDT=off  OutDataTypeStr=boolean
  XOR1 : Logic  Operator=XOR  IconShape=distinctive  AllPortsSameDT=off  OutDataTypeStr=boolean
  Sum : Outport
  Carry : Outport  Port=2
  wires:
  SumIn/1 -> XOR1/1, AND/1
  XOR1/1 -> AND1/1, XOR/1
  Cin/1 -> XOR/2, AND1/2
  XOR/1 -> Sum/1
  AND2/1 -> AND/2, XOR1/2
  "OR "/1 -> Carry/1
  AND1/1 -> "OR "/1
  AND/1 -> "OR "/2
  B/1 -> AND2/2
  A/1 -> AND2/1

== system ExtraCredit/Subsystem/Subsystem/MultiBlock23 ==
  SumIn : Inport
  Cin : Inport  Port=2
  B : Inport  Port=3
  A : Inport  Port=4
  AND : Logic  IconShape=distinctive  AllPortsSameDT=off  OutDataTypeStr=boolean
  AND1 : Logic  IconShape=distinctive  AllPortsSameDT=off  OutDataTypeStr=boolean
  AND2 : Logic  IconShape=distinctive  AllPortsSameDT=off  OutDataTypeStr=boolean
  "OR " : Logic  Operator=OR  IconShape=distinctive  AllPortsSameDT=off  OutDataTypeStr=boolean
  XOR : Logic  Operator=XOR  IconShape=distinctive  AllPortsSameDT=off  OutDataTypeStr=boolean
  XOR1 : Logic  Operator=XOR  IconShape=distinctive  AllPortsSameDT=off  OutDataTypeStr=boolean
  Sum : Outport
  Carry : Outport  Port=2
  wires:
  SumIn/1 -> XOR1/1, AND/1
  XOR1/1 -> AND1/1, XOR/1
  Cin/1 -> XOR/2, AND1/2
  XOR/1 -> Sum/1
  AND2/1 -> AND/2, XOR1/2
  "OR "/1 -> Carry/1
  AND1/1 -> "OR "/1
  AND/1 -> "OR "/2
  B/1 -> AND2/2
  A/1 -> AND2/1

== system ExtraCredit/Subsystem/Subsystem/MultiBlock24 ==
  SumIn : Inport
  Cin : Inport  Port=2
  B : Inport  Port=3
  A : Inport  Port=4
  AND : Logic  IconShape=distinctive  AllPortsSameDT=off  OutDataTypeStr=boolean
  AND1 : Logic  IconShape=distinctive  AllPortsSameDT=off  OutDataTypeStr=boolean
  AND2 : Logic  IconShape=distinctive  AllPortsSameDT=off  OutDataTypeStr=boolean
  "OR " : Logic  Operator=OR  IconShape=distinctive  AllPortsSameDT=off  OutDataTypeStr=boolean
  XOR : Logic  Operator=XOR  IconShape=distinctive  AllPortsSameDT=off  OutDataTypeStr=boolean
  XOR1 : Logic  Operator=XOR  IconShape=distinctive  AllPortsSameDT=off  OutDataTypeStr=boolean
  Sum : Outport
  Carry : Outport  Port=2
  wires:
  SumIn/1 -> XOR1/1, AND/1
  XOR1/1 -> AND1/1, XOR/1
  Cin/1 -> XOR/2, AND1/2
  XOR/1 -> Sum/1
  AND2/1 -> AND/2, XOR1/2
  "OR "/1 -> Carry/1
  AND1/1 -> "OR "/1
  AND/1 -> "OR "/2
  B/1 -> AND2/2
  A/1 -> AND2/1

== system ExtraCredit/Subsystem/Subsystem/MultiBlock25 ==
  SumIn : Inport
  Cin : Inport  Port=2
  B : Inport  Port=3
  A : Inport  Port=4
  AND : Logic  IconShape=distinctive  AllPortsSameDT=off  OutDataTypeStr=boolean
  AND1 : Logic  IconShape=distinctive  AllPortsSameDT=off  OutDataTypeStr=boolean
  AND2 : Logic  IconShape=distinctive  AllPortsSameDT=off  OutDataTypeStr=boolean
  "OR " : Logic  Operator=OR  IconShape=distinctive  AllPortsSameDT=off  OutDataTypeStr=boolean
  XOR : Logic  Operator=XOR  IconShape=distinctive  AllPortsSameDT=off  OutDataTypeStr=boolean
  XOR1 : Logic  Operator=XOR  IconShape=distinctive  AllPortsSameDT=off  OutDataTypeStr=boolean
  Sum : Outport
  Carry : Outport  Port=2
  wires:
  SumIn/1 -> XOR1/1, AND/1
  XOR1/1 -> AND1/1, XOR/1
  Cin/1 -> XOR/2, AND1/2
  XOR/1 -> Sum/1
  AND2/1 -> AND/2, XOR1/2
  "OR "/1 -> Carry/1
  AND1/1 -> "OR "/1
  AND/1 -> "OR "/2
  B/1 -> AND2/2
  A/1 -> AND2/1

== system ExtraCredit/Subsystem/Subsystem/MultiBlock26 ==
  SumIn : Inport
  Cin : Inport  Port=2
  B : Inport  Port=3
  A : Inport  Port=4
  AND : Logic  IconShape=distinctive  AllPortsSameDT=off  OutDataTypeStr=boolean
  AND1 : Logic  IconShape=distinctive  AllPortsSameDT=off  OutDataTypeStr=boolean
  AND2 : Logic  IconShape=distinctive  AllPortsSameDT=off  OutDataTypeStr=boolean
  "OR " : Logic  Operator=OR  IconShape=distinctive  AllPortsSameDT=off  OutDataTypeStr=boolean
  XOR : Logic  Operator=XOR  IconShape=distinctive  AllPortsSameDT=off  OutDataTypeStr=boolean
  XOR1 : Logic  Operator=XOR  IconShape=distinctive  AllPortsSameDT=off  OutDataTypeStr=boolean
  Sum : Outport
  Carry : Outport  Port=2
  wires:
  SumIn/1 -> XOR1/1, AND/1
  XOR1/1 -> AND1/1, XOR/1
  Cin/1 -> XOR/2, AND1/2
  XOR/1 -> Sum/1
  AND2/1 -> AND/2, XOR1/2
  "OR "/1 -> Carry/1
  AND1/1 -> "OR "/1
  AND/1 -> "OR "/2
  B/1 -> AND2/2
  A/1 -> AND2/1

== system ExtraCredit/Subsystem/Subsystem/MultiBlock27 ==
  SumIn : Inport
  Cin : Inport  Port=2
  B : Inport  Port=3
  A : Inport  Port=4
  AND : Logic  IconShape=distinctive  AllPortsSameDT=off  OutDataTypeStr=boolean
  AND1 : Logic  IconShape=distinctive  AllPortsSameDT=off  OutDataTypeStr=boolean
  AND2 : Logic  IconShape=distinctive  AllPortsSameDT=off  OutDataTypeStr=boolean
  "OR " : Logic  Operator=OR  IconShape=distinctive  AllPortsSameDT=off  OutDataTypeStr=boolean
  XOR : Logic  Operator=XOR  IconShape=distinctive  AllPortsSameDT=off  OutDataTypeStr=boolean
  XOR1 : Logic  Operator=XOR  IconShape=distinctive  AllPortsSameDT=off  OutDataTypeStr=boolean
  Sum : Outport
  Carry : Outport  Port=2
  wires:
  SumIn/1 -> XOR1/1, AND/1
  XOR1/1 -> AND1/1, XOR/1
  Cin/1 -> XOR/2, AND1/2
  XOR/1 -> Sum/1
  AND2/1 -> AND/2, XOR1/2
  "OR "/1 -> Carry/1
  AND1/1 -> "OR "/1
  AND/1 -> "OR "/2
  B/1 -> AND2/2
  A/1 -> AND2/1

== system ExtraCredit/Subsystem/Subsystem/MultiBlock28 ==
  SumIn : Inport
  Cin : Inport  Port=2
  B : Inport  Port=3
  A : Inport  Port=4
  AND : Logic  IconShape=distinctive  AllPortsSameDT=off  OutDataTypeStr=boolean
  AND1 : Logic  IconShape=distinctive  AllPortsSameDT=off  OutDataTypeStr=boolean
  AND2 : Logic  IconShape=distinctive  AllPortsSameDT=off  OutDataTypeStr=boolean
  "OR " : Logic  Operator=OR  IconShape=distinctive  AllPortsSameDT=off  OutDataTypeStr=boolean
  XOR : Logic  Operator=XOR  IconShape=distinctive  AllPortsSameDT=off  OutDataTypeStr=boolean
  XOR1 : Logic  Operator=XOR  IconShape=distinctive  AllPortsSameDT=off  OutDataTypeStr=boolean
  Sum : Outport
  Carry : Outport  Port=2
  wires:
  SumIn/1 -> XOR1/1, AND/1
  XOR1/1 -> AND1/1, XOR/1
  Cin/1 -> XOR/2, AND1/2
  XOR/1 -> Sum/1
  AND2/1 -> AND/2, XOR1/2
  "OR "/1 -> Carry/1
  AND1/1 -> "OR "/1
  AND/1 -> "OR "/2
  B/1 -> AND2/2
  A/1 -> AND2/1

== system ExtraCredit/Subsystem/Subsystem/MultiBlock29 ==
  SumIn : Inport
  Cin : Inport  Port=2
  B : Inport  Port=3
  A : Inport  Port=4
  AND : Logic  IconShape=distinctive  AllPortsSameDT=off  OutDataTypeStr=boolean
  AND1 : Logic  IconShape=distinctive  AllPortsSameDT=off  OutDataTypeStr=boolean
  AND2 : Logic  IconShape=distinctive  AllPortsSameDT=off  OutDataTypeStr=boolean
  "OR " : Logic  Operator=OR  IconShape=distinctive  AllPortsSameDT=off  OutDataTypeStr=boolean
  XOR : Logic  Operator=XOR  IconShape=distinctive  AllPortsSameDT=off  OutDataTypeStr=boolean
  XOR1 : Logic  Operator=XOR  IconShape=distinctive  AllPortsSameDT=off  OutDataTypeStr=boolean
  Sum : Outport
  Carry : Outport  Port=2
  wires:
  SumIn/1 -> XOR1/1, AND/1
  XOR1/1 -> AND1/1, XOR/1
  Cin/1 -> XOR/2, AND1/2
  XOR/1 -> Sum/1
  AND2/1 -> AND/2, XOR1/2
  "OR "/1 -> Carry/1
  AND1/1 -> "OR "/1
  AND/1 -> "OR "/2
  B/1 -> AND2/2
  A/1 -> AND2/1

== system ExtraCredit/Subsystem/Subsystem/MultiBlock3 ==
  SumIn : Inport
  Cin : Inport  Port=2
  B : Inport  Port=3
  A : Inport  Port=4
  AND : Logic  IconShape=distinctive  AllPortsSameDT=off  OutDataTypeStr=boolean
  AND1 : Logic  IconShape=distinctive  AllPortsSameDT=off  OutDataTypeStr=boolean
  AND2 : Logic  IconShape=distinctive  AllPortsSameDT=off  OutDataTypeStr=boolean
  "OR " : Logic  Operator=OR  IconShape=distinctive  AllPortsSameDT=off  OutDataTypeStr=boolean
  XOR : Logic  Operator=XOR  IconShape=distinctive  AllPortsSameDT=off  OutDataTypeStr=boolean
  XOR1 : Logic  Operator=XOR  IconShape=distinctive  AllPortsSameDT=off  OutDataTypeStr=boolean
  Sum : Outport
  Carry : Outport  Port=2
  wires:
  SumIn/1 -> XOR1/1, AND/1
  XOR1/1 -> AND1/1, XOR/1
  Cin/1 -> XOR/2, AND1/2
  XOR/1 -> Sum/1
  AND2/1 -> AND/2, XOR1/2
  "OR "/1 -> Carry/1
  AND1/1 -> "OR "/1
  AND/1 -> "OR "/2
  B/1 -> AND2/2
  A/1 -> AND2/1

== system ExtraCredit/Subsystem/Subsystem/MultiBlock30 ==
  SumIn : Inport
  Cin : Inport  Port=2
  B : Inport  Port=3
  A : Inport  Port=4
  AND : Logic  IconShape=distinctive  AllPortsSameDT=off  OutDataTypeStr=boolean
  AND1 : Logic  IconShape=distinctive  AllPortsSameDT=off  OutDataTypeStr=boolean
  AND2 : Logic  IconShape=distinctive  AllPortsSameDT=off  OutDataTypeStr=boolean
  "OR " : Logic  Operator=OR  IconShape=distinctive  AllPortsSameDT=off  OutDataTypeStr=boolean
  XOR : Logic  Operator=XOR  IconShape=distinctive  AllPortsSameDT=off  OutDataTypeStr=boolean
  XOR1 : Logic  Operator=XOR  IconShape=distinctive  AllPortsSameDT=off  OutDataTypeStr=boolean
  Sum : Outport
  Carry : Outport  Port=2
  wires:
  SumIn/1 -> XOR1/1, AND/1
  XOR1/1 -> AND1/1, XOR/1
  Cin/1 -> XOR/2, AND1/2
  XOR/1 -> Sum/1
  AND2/1 -> AND/2, XOR1/2
  "OR "/1 -> Carry/1
  AND1/1 -> "OR "/1
  AND/1 -> "OR "/2
  B/1 -> AND2/2
  A/1 -> AND2/1

== system ExtraCredit/Subsystem/Subsystem/MultiBlock31 ==
  SumIn : Inport
  Cin : Inport  Port=2
  B : Inport  Port=3
  A : Inport  Port=4
  AND : Logic  IconShape=distinctive  AllPortsSameDT=off  OutDataTypeStr=boolean
  AND1 : Logic  IconShape=distinctive  AllPortsSameDT=off  OutDataTypeStr=boolean
  AND2 : Logic  IconShape=distinctive  AllPortsSameDT=off  OutDataTypeStr=boolean
  "OR " : Logic  Operator=OR  IconShape=distinctive  AllPortsSameDT=off  OutDataTypeStr=boolean
  XOR : Logic  Operator=XOR  IconShape=distinctive  AllPortsSameDT=off  OutDataTypeStr=boolean
  XOR1 : Logic  Operator=XOR  IconShape=distinctive  AllPortsSameDT=off  OutDataTypeStr=boolean
  Sum : Outport
  Carry : Outport  Port=2
  wires:
  SumIn/1 -> XOR1/1, AND/1
  XOR1/1 -> AND1/1, XOR/1
  Cin/1 -> XOR/2, AND1/2
  XOR/1 -> Sum/1
  AND2/1 -> AND/2, XOR1/2
  "OR "/1 -> Carry/1
  AND1/1 -> "OR "/1
  AND/1 -> "OR "/2
  B/1 -> AND2/2
  A/1 -> AND2/1

== system ExtraCredit/Subsystem/Subsystem/MultiBlock32 ==
  SumIn : Inport
  Cin : Inport  Port=2
  B : Inport  Port=3
  A : Inport  Port=4
  AND : Logic  IconShape=distinctive  AllPortsSameDT=off  OutDataTypeStr=boolean
  AND1 : Logic  IconShape=distinctive  AllPortsSameDT=off  OutDataTypeStr=boolean
  AND2 : Logic  IconShape=distinctive  AllPortsSameDT=off  OutDataTypeStr=boolean
  "OR " : Logic  Operator=OR  IconShape=distinctive  AllPortsSameDT=off  OutDataTypeStr=boolean
  XOR : Logic  Operator=XOR  IconShape=distinctive  AllPortsSameDT=off  OutDataTypeStr=boolean
  XOR1 : Logic  Operator=XOR  IconShape=distinctive  AllPortsSameDT=off  OutDataTypeStr=boolean
  Sum : Outport
  Carry : Outport  Port=2
  wires:
  SumIn/1 -> XOR1/1, AND/1
  XOR1/1 -> AND1/1, XOR/1
  Cin/1 -> XOR/2, AND1/2
  XOR/1 -> Sum/1
  AND2/1 -> AND/2, XOR1/2
  "OR "/1 -> Carry/1
  AND1/1 -> "OR "/1
  AND/1 -> "OR "/2
  B/1 -> AND2/2
  A/1 -> AND2/1

== system ExtraCredit/Subsystem/Subsystem/MultiBlock33 ==
  SumIn : Inport
  Cin : Inport  Port=2
  B : Inport  Port=3
  A : Inport  Port=4
  AND : Logic  IconShape=distinctive  AllPortsSameDT=off  OutDataTypeStr=boolean
  AND1 : Logic  IconShape=distinctive  AllPortsSameDT=off  OutDataTypeStr=boolean
  AND2 : Logic  IconShape=distinctive  AllPortsSameDT=off  OutDataTypeStr=boolean
  "OR " : Logic  Operator=OR  IconShape=distinctive  AllPortsSameDT=off  OutDataTypeStr=boolean
  XOR : Logic  Operator=XOR  IconShape=distinctive  AllPortsSameDT=off  OutDataTypeStr=boolean
  XOR1 : Logic  Operator=XOR  IconShape=distinctive  AllPortsSameDT=off  OutDataTypeStr=boolean
  Sum : Outport
  Carry : Outport  Port=2
  wires:
  SumIn/1 -> XOR1/1, AND/1
  XOR1/1 -> AND1/1, XOR/1
  Cin/1 -> XOR/2, AND1/2
  XOR/1 -> Sum/1
  AND2/1 -> AND/2, XOR1/2
  "OR "/1 -> Carry/1
  AND1/1 -> "OR "/1
  AND/1 -> "OR "/2
  B/1 -> AND2/2
  A/1 -> AND2/1

== system ExtraCredit/Subsystem/Subsystem/MultiBlock34 ==
  SumIn : Inport
  Cin : Inport  Port=2
  B : Inport  Port=3
  A : Inport  Port=4
  AND : Logic  IconShape=distinctive  AllPortsSameDT=off  OutDataTypeStr=boolean
  AND1 : Logic  IconShape=distinctive  AllPortsSameDT=off  OutDataTypeStr=boolean
  AND2 : Logic  IconShape=distinctive  AllPortsSameDT=off  OutDataTypeStr=boolean
  "OR " : Logic  Operator=OR  IconShape=distinctive  AllPortsSameDT=off  OutDataTypeStr=boolean
  XOR : Logic  Operator=XOR  IconShape=distinctive  AllPortsSameDT=off  OutDataTypeStr=boolean
  XOR1 : Logic  Operator=XOR  IconShape=distinctive  AllPortsSameDT=off  OutDataTypeStr=boolean
  Sum : Outport
  Carry : Outport  Port=2
  wires:
  SumIn/1 -> XOR1/1, AND/1
  XOR1/1 -> AND1/1, XOR/1
  Cin/1 -> XOR/2, AND1/2
  XOR/1 -> Sum/1
  AND2/1 -> AND/2, XOR1/2
  "OR "/1 -> Carry/1
  AND1/1 -> "OR "/1
  AND/1 -> "OR "/2
  B/1 -> AND2/2
  A/1 -> AND2/1

== system ExtraCredit/Subsystem/Subsystem/MultiBlock35 ==
  SumIn : Inport
  Cin : Inport  Port=2
  B : Inport  Port=3
  A : Inport  Port=4
  AND : Logic  IconShape=distinctive  AllPortsSameDT=off  OutDataTypeStr=boolean
  AND1 : Logic  IconShape=distinctive  AllPortsSameDT=off  OutDataTypeStr=boolean
  AND2 : Logic  IconShape=distinctive  AllPortsSameDT=off  OutDataTypeStr=boolean
  "OR " : Logic  Operator=OR  IconShape=distinctive  AllPortsSameDT=off  OutDataTypeStr=boolean
  XOR : Logic  Operator=XOR  IconShape=distinctive  AllPortsSameDT=off  OutDataTypeStr=boolean
  XOR1 : Logic  Operator=XOR  IconShape=distinctive  AllPortsSameDT=off  OutDataTypeStr=boolean
  Sum : Outport
  Carry : Outport  Port=2
  wires:
  SumIn/1 -> XOR1/1, AND/1
  XOR1/1 -> AND1/1, XOR/1
  Cin/1 -> XOR/2, AND1/2
  XOR/1 -> Sum/1
  AND2/1 -> AND/2, XOR1/2
  "OR "/1 -> Carry/1
  AND1/1 -> "OR "/1
  AND/1 -> "OR "/2
  B/1 -> AND2/2
  A/1 -> AND2/1

== system ExtraCredit/Subsystem/Subsystem/MultiBlock36 ==
  SumIn : Inport
  Cin : Inport  Port=2
  B : Inport  Port=3
  A : Inport  Port=4
  AND : Logic  IconShape=distinctive  AllPortsSameDT=off  OutDataTypeStr=boolean
  AND1 : Logic  IconShape=distinctive  AllPortsSameDT=off  OutDataTypeStr=boolean
  AND2 : Logic  IconShape=distinctive  AllPortsSameDT=off  OutDataTypeStr=boolean
  "OR " : Logic  Operator=OR  IconShape=distinctive  AllPortsSameDT=off  OutDataTypeStr=boolean
  XOR : Logic  Operator=XOR  IconShape=distinctive  AllPortsSameDT=off  OutDataTypeStr=boolean
  XOR1 : Logic  Operator=XOR  IconShape=distinctive  AllPortsSameDT=off  OutDataTypeStr=boolean
  Sum : Outport
  Carry : Outport  Port=2
  wires:
  SumIn/1 -> XOR1/1, AND/1
  XOR1/1 -> AND1/1, XOR/1
  Cin/1 -> XOR/2, AND1/2
  XOR/1 -> Sum/1
  AND2/1 -> AND/2, XOR1/2
  "OR "/1 -> Carry/1
  AND1/1 -> "OR "/1
  AND/1 -> "OR "/2
  B/1 -> AND2/2
  A/1 -> AND2/1

== system ExtraCredit/Subsystem/Subsystem/MultiBlock37 ==
  SumIn : Inport
  Cin : Inport  Port=2
  B : Inport  Port=3
  A : Inport  Port=4
  AND : Logic  IconShape=distinctive  AllPortsSameDT=off  OutDataTypeStr=boolean
  AND1 : Logic  IconShape=distinctive  AllPortsSameDT=off  OutDataTypeStr=boolean
  AND2 : Logic  IconShape=distinctive  AllPortsSameDT=off  OutDataTypeStr=boolean
  "OR " : Logic  Operator=OR  IconShape=distinctive  AllPortsSameDT=off  OutDataTypeStr=boolean
  XOR : Logic  Operator=XOR  IconShape=distinctive  AllPortsSameDT=off  OutDataTypeStr=boolean
  XOR1 : Logic  Operator=XOR  IconShape=distinctive  AllPortsSameDT=off  OutDataTypeStr=boolean
  Sum : Outport
  Carry : Outport  Port=2
  wires:
  SumIn/1 -> XOR1/1, AND/1
  XOR1/1 -> AND1/1, XOR/1
  Cin/1 -> XOR/2, AND1/2
  XOR/1 -> Sum/1
  AND2/1 -> AND/2, XOR1/2
  "OR "/1 -> Carry/1
  AND1/1 -> "OR "/1
  AND/1 -> "OR "/2
  B/1 -> AND2/2
  A/1 -> AND2/1

== system ExtraCredit/Subsystem/Subsystem/MultiBlock38 ==
  SumIn : Inport
  Cin : Inport  Port=2
  B : Inport  Port=3
  A : Inport  Port=4
  AND : Logic  IconShape=distinctive  AllPortsSameDT=off  OutDataTypeStr=boolean
  AND1 : Logic  IconShape=distinctive  AllPortsSameDT=off  OutDataTypeStr=boolean
  AND2 : Logic  IconShape=distinctive  AllPortsSameDT=off  OutDataTypeStr=boolean
  "OR " : Logic  Operator=OR  IconShape=distinctive  AllPortsSameDT=off  OutDataTypeStr=boolean
  XOR : Logic  Operator=XOR  IconShape=distinctive  AllPortsSameDT=off  OutDataTypeStr=boolean
  XOR1 : Logic  Operator=XOR  IconShape=distinctive  AllPortsSameDT=off  OutDataTypeStr=boolean
  Sum : Outport
  Carry : Outport  Port=2
  wires:
  SumIn/1 -> XOR1/1, AND/1
  XOR1/1 -> AND1/1, XOR/1
  Cin/1 -> XOR/2, AND1/2
  XOR/1 -> Sum/1
  AND2/1 -> AND/2, XOR1/2
  "OR "/1 -> Carry/1
  AND1/1 -> "OR "/1
  AND/1 -> "OR "/2
  B/1 -> AND2/2
  A/1 -> AND2/1

== system ExtraCredit/Subsystem/Subsystem/MultiBlock39 ==
  SumIn : Inport
  Cin : Inport  Port=2
  B : Inport  Port=3
  A : Inport  Port=4
  AND : Logic  IconShape=distinctive  AllPortsSameDT=off  OutDataTypeStr=boolean
  AND1 : Logic  IconShape=distinctive  AllPortsSameDT=off  OutDataTypeStr=boolean
  AND2 : Logic  IconShape=distinctive  AllPortsSameDT=off  OutDataTypeStr=boolean
  "OR " : Logic  Operator=OR  IconShape=distinctive  AllPortsSameDT=off  OutDataTypeStr=boolean
  XOR : Logic  Operator=XOR  IconShape=distinctive  AllPortsSameDT=off  OutDataTypeStr=boolean
  XOR1 : Logic  Operator=XOR  IconShape=distinctive  AllPortsSameDT=off  OutDataTypeStr=boolean
  Sum : Outport
  Carry : Outport  Port=2
  wires:
  SumIn/1 -> XOR1/1, AND/1
  XOR1/1 -> AND1/1, XOR/1
  Cin/1 -> XOR/2, AND1/2
  XOR/1 -> Sum/1
  AND2/1 -> AND/2, XOR1/2
  "OR "/1 -> Carry/1
  AND1/1 -> "OR "/1
  AND/1 -> "OR "/2
  B/1 -> AND2/2
  A/1 -> AND2/1

== system ExtraCredit/Subsystem/Subsystem/MultiBlock4 ==
  SumIn : Inport
  Cin : Inport  Port=2
  B : Inport  Port=3
  A : Inport  Port=4
  AND : Logic  IconShape=distinctive  AllPortsSameDT=off  OutDataTypeStr=boolean
  AND1 : Logic  IconShape=distinctive  AllPortsSameDT=off  OutDataTypeStr=boolean
  AND2 : Logic  IconShape=distinctive  AllPortsSameDT=off  OutDataTypeStr=boolean
  "OR " : Logic  Operator=OR  IconShape=distinctive  AllPortsSameDT=off  OutDataTypeStr=boolean
  XOR : Logic  Operator=XOR  IconShape=distinctive  AllPortsSameDT=off  OutDataTypeStr=boolean
  XOR1 : Logic  Operator=XOR  IconShape=distinctive  AllPortsSameDT=off  OutDataTypeStr=boolean
  Sum : Outport
  Carry : Outport  Port=2
  wires:
  SumIn/1 -> XOR1/1, AND/1
  XOR1/1 -> AND1/1, XOR/1
  Cin/1 -> XOR/2, AND1/2
  XOR/1 -> Sum/1
  AND2/1 -> AND/2, XOR1/2
  "OR "/1 -> Carry/1
  AND1/1 -> "OR "/1
  AND/1 -> "OR "/2
  B/1 -> AND2/2
  A/1 -> AND2/1

== system ExtraCredit/Subsystem/Subsystem/MultiBlock40 ==
  SumIn : Inport
  Cin : Inport  Port=2
  B : Inport  Port=3
  A : Inport  Port=4
  AND : Logic  IconShape=distinctive  AllPortsSameDT=off  OutDataTypeStr=boolean
  AND1 : Logic  IconShape=distinctive  AllPortsSameDT=off  OutDataTypeStr=boolean
  AND2 : Logic  IconShape=distinctive  AllPortsSameDT=off  OutDataTypeStr=boolean
  "OR " : Logic  Operator=OR  IconShape=distinctive  AllPortsSameDT=off  OutDataTypeStr=boolean
  XOR : Logic  Operator=XOR  IconShape=distinctive  AllPortsSameDT=off  OutDataTypeStr=boolean
  XOR1 : Logic  Operator=XOR  IconShape=distinctive  AllPortsSameDT=off  OutDataTypeStr=boolean
  Sum : Outport
  Carry : Outport  Port=2
  wires:
  SumIn/1 -> XOR1/1, AND/1
  XOR1/1 -> AND1/1, XOR/1
  Cin/1 -> XOR/2, AND1/2
  XOR/1 -> Sum/1
  AND2/1 -> AND/2, XOR1/2
  "OR "/1 -> Carry/1
  AND1/1 -> "OR "/1
  AND/1 -> "OR "/2
  B/1 -> AND2/2
  A/1 -> AND2/1

== system ExtraCredit/Subsystem/Subsystem/MultiBlock41 ==
  SumIn : Inport
  Cin : Inport  Port=2
  B : Inport  Port=3
  A : Inport  Port=4
  AND : Logic  IconShape=distinctive  AllPortsSameDT=off  OutDataTypeStr=boolean
  AND1 : Logic  IconShape=distinctive  AllPortsSameDT=off  OutDataTypeStr=boolean
  AND2 : Logic  IconShape=distinctive  AllPortsSameDT=off  OutDataTypeStr=boolean
  "OR " : Logic  Operator=OR  IconShape=distinctive  AllPortsSameDT=off  OutDataTypeStr=boolean
  XOR : Logic  Operator=XOR  IconShape=distinctive  AllPortsSameDT=off  OutDataTypeStr=boolean
  XOR1 : Logic  Operator=XOR  IconShape=distinctive  AllPortsSameDT=off  OutDataTypeStr=boolean
  Sum : Outport
  Carry : Outport  Port=2
  wires:
  SumIn/1 -> XOR1/1, AND/1
  XOR1/1 -> AND1/1, XOR/1
  Cin/1 -> XOR/2, AND1/2
  XOR/1 -> Sum/1
  AND2/1 -> AND/2, XOR1/2
  "OR "/1 -> Carry/1
  AND1/1 -> "OR "/1
  AND/1 -> "OR "/2
  B/1 -> AND2/2
  A/1 -> AND2/1

== system ExtraCredit/Subsystem/Subsystem/MultiBlock42 ==
  SumIn : Inport
  Cin : Inport  Port=2
  B : Inport  Port=3
  A : Inport  Port=4
  AND : Logic  IconShape=distinctive  AllPortsSameDT=off  OutDataTypeStr=boolean
  AND1 : Logic  IconShape=distinctive  AllPortsSameDT=off  OutDataTypeStr=boolean
  AND2 : Logic  IconShape=distinctive  AllPortsSameDT=off  OutDataTypeStr=boolean
  "OR " : Logic  Operator=OR  IconShape=distinctive  AllPortsSameDT=off  OutDataTypeStr=boolean
  XOR : Logic  Operator=XOR  IconShape=distinctive  AllPortsSameDT=off  OutDataTypeStr=boolean
  XOR1 : Logic  Operator=XOR  IconShape=distinctive  AllPortsSameDT=off  OutDataTypeStr=boolean
  Sum : Outport
  Carry : Outport  Port=2
  wires:
  SumIn/1 -> XOR1/1, AND/1
  XOR1/1 -> AND1/1, XOR/1
  Cin/1 -> XOR/2, AND1/2
  XOR/1 -> Sum/1
  AND2/1 -> AND/2, XOR1/2
  "OR "/1 -> Carry/1
  AND1/1 -> "OR "/1
  AND/1 -> "OR "/2
  B/1 -> AND2/2
  A/1 -> AND2/1

== system ExtraCredit/Subsystem/Subsystem/MultiBlock43 ==
  SumIn : Inport
  Cin : Inport  Port=2
  B : Inport  Port=3
  A : Inport  Port=4
  AND : Logic  IconShape=distinctive  AllPortsSameDT=off  OutDataTypeStr=boolean
  AND1 : Logic  IconShape=distinctive  AllPortsSameDT=off  OutDataTypeStr=boolean
  AND2 : Logic  IconShape=distinctive  AllPortsSameDT=off  OutDataTypeStr=boolean
  "OR " : Logic  Operator=OR  IconShape=distinctive  AllPortsSameDT=off  OutDataTypeStr=boolean
  XOR : Logic  Operator=XOR  IconShape=distinctive  AllPortsSameDT=off  OutDataTypeStr=boolean
  XOR1 : Logic  Operator=XOR  IconShape=distinctive  AllPortsSameDT=off  OutDataTypeStr=boolean
  Sum : Outport
  Carry : Outport  Port=2
  wires:
  SumIn/1 -> XOR1/1, AND/1
  XOR1/1 -> AND1/1, XOR/1
  Cin/1 -> XOR/2, AND1/2
  XOR/1 -> Sum/1
  AND2/1 -> AND/2, XOR1/2
  "OR "/1 -> Carry/1
  AND1/1 -> "OR "/1
  AND/1 -> "OR "/2
  B/1 -> AND2/2
  A/1 -> AND2/1
